simulink model "check_ndtm_poweroversteer"  (R2018b)
settings: configuration reference "Physics" (kept outside this file)
settings Model: DataDictionary=check_ndtm.sldd  OrderedModelArguments=off  Creator=wischnewski  LastModifiedBy=ga25xiw

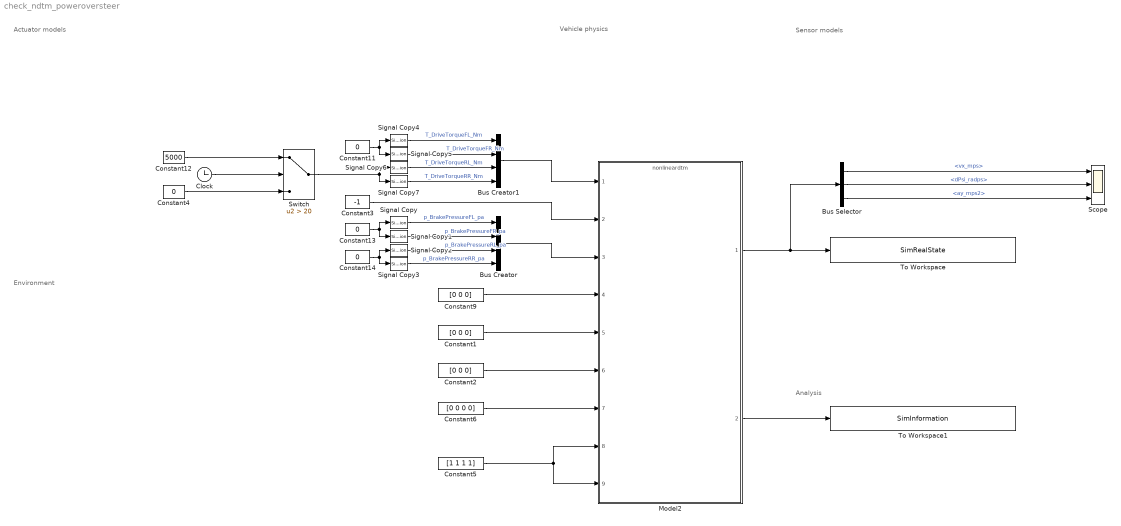
== system check_ndtm_poweroversteer ==
  note: Actuator models
  note: Vehicle physics
  note: Environment
  note: Analysis
  note: Sensor models
  Bus Creator : BusCreator  Inputs=4  OutDataTypeStr=Bus: BrakePressure_Pa
  Bus Creator1 : BusCreator  Inputs=4  OutDataTypeStr=Bus: DriveTorque_Nm
  Bus Selector : BusSelector  OutputSignals=vx_mps,dPsi_radps,ay_mps2
  Clock : Clock
  Constant1 : Constant  Value=[0 0 0]
  Constant{4,11,13..14} (4 alike) : Constant  Value=0
  Constant12 : Constant  Value=5000
  Constant2 : Constant  Value=[0 0 0]
  Constant3 : Constant  Value=-1
  Constant5 : Constant  Value=[1 1 1 1]
  Constant6 : Constant  Value=[0 0 0 0]
  Constant9 : Constant  Value=[0 0 0]
  Model2 : ModelReference  ModelNameDialog=nonlineardtm  ParameterArgumentNames=x0_initialstates  ParameterArgumentValues=[0 0 0 0 0 -pi/2]  UsingDefaultArgumentValue=0  SimulationMode=Normal  ModelReferenceVersion=1.642
  Scope : Scope  NumInputPorts=3
  Signal Copy{,1..7} (8 alike) : SignalConversion  OverrideOpt=off
  Switch : Switch  Criteria=u2 > Threshold  Threshold=20
  To Workspace : ToWorkspace  VariableName=SimRealState  SaveFormat=Timeseries  SampleTime=-1
  To Workspace1 : ToWorkspace  VariableName=SimInformation  SaveFormat=Timeseries  SampleTime=-1
  wires:
  Bus Selector/1 -> Scope/1  "<vx_mps>"
  Bus Selector/2 -> Scope/2  "<dPsi_radps>"
  Bus Selector/3 -> Scope/3  "<ay_mps2>"
  Model2/1 -> Bus Selector/1, To Workspace/1
  Constant9/1 -> Model2/4
  Constant1/1 -> Model2/5
  Constant2/1 -> Model2/6
  Constant5/1 -> Model2/9, Model2/8
  Constant6/1 -> Model2/7
  Model2/2 -> To Workspace1/1
  Constant11/1 -> Signal Copy4/1, Signal Copy5/1
  Signal Copy6/1 -> Bus Creator1/3  "T_DriveTorqueRL_Nm"
  Signal Copy5/1 -> Bus Creator1/2  "T_DriveTorqueFR_Nm"
  Signal Copy7/1 -> Bus Creator1/4  "T_DriveTorqueRR_Nm"
  Signal Copy4/1 -> Bus Creator1/1  "T_DriveTorqueFL_Nm"
  Bus Creator1/1 -> Model2/1
  Constant14/1 -> Signal Copy3/1, Signal Copy2/1
  Constant13/1 -> Signal Copy1/1, Signal Copy/1
  Signal Copy2/1 -> Bus Creator/3  "p_BrakePressureRL_pa"
  Signal Copy1/1 -> Bus Creator/2  "p_BrakePressureFR_pa"
  Switch/1 -> Signal Copy6/1, Signal Copy7/1
  Bus Creator/1 -> Model2/3
  Constant3/1 -> Model2/2
  Signal Copy3/1 -> Bus Creator/4  "p_BrakePressureRR_pa"
  Signal Copy/1 -> Bus Creator/1  "p_BrakePressureFL_pa"
  Clock/1 -> Switch/2
  Constant4/1 -> Switch/3
  Constant12/1 -> Switch/1
